simulink model "Torque_controller_MIL"  (R2023b)
settings: Solver=VariableStepAuto  StartTime=0.0  StopTime=15  RelTol=1e-3
values from neighbouring files (symbols this model uses):
  b = 0.016*2.5    (= 0.04)    [torque.m]
  Im = 0.0059*10    (= 0.059)    [torque.m]
  k = kt    (= 1.45433391507)    [torque.m]
  L = 0.0472    [torque.m]
  R = 2.0    (= 2)    [torque.m]
  Ts = 0.005    [torque.m]
libraries: cstblocks x3, simulink x1
settings Model: Creator=giova  LastModifiedBy=david

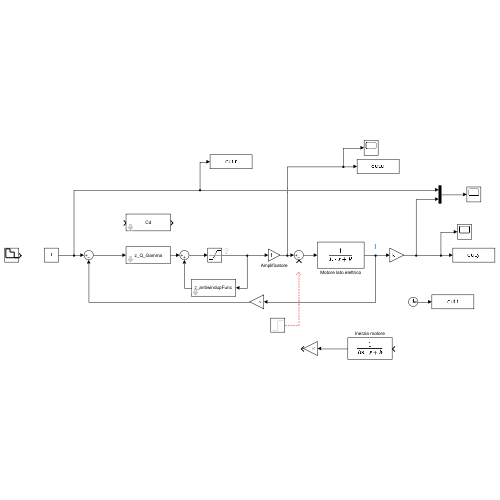
[thumbnail: Simulink's stored preview of the top-level diagram]
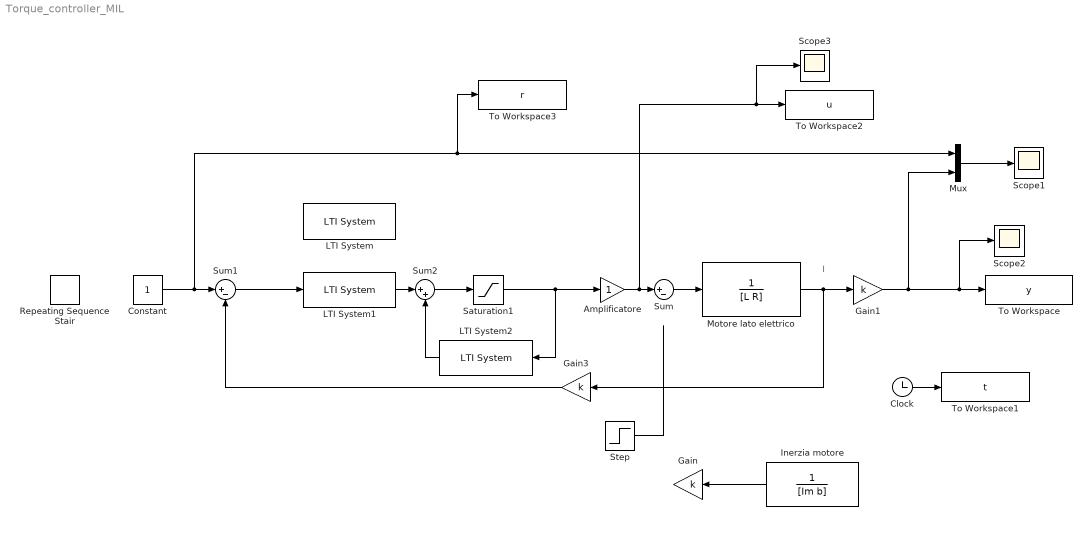
== system Torque_controller_MIL ==
  note: I
  Amplificatore : Gain
  Clock : Clock
  Constant : Constant
  Gain : Gain  Gain=k
  Gain1 : Gain  Gain=k
  Gain3 : Gain  Gain=k
  Inerzia motore : TransferFcn  Denominator=[Im b]
  LTI System : cstblocks/LTI System  sys=Cd  IC=[]  PadeOrder=0
  LTI System1 : cstblocks/LTI System  sys=z_Q_Gamma  IC=[]  PadeOrder=0
  LTI System2 : cstblocks/LTI System  sys=z_antiwindupFunc  IC=[]  PadeOrder=0
  Motore lato elettrico : TransferFcn  Denominator=[L R]
  Mux : Mux  Inputs=2
  Repeating Sequence Stair : simulink/Sources/Repeating Sequence Stair  OutValues=[0.32 0.2 0]  tsamp=5  OutMin=[]  OutMax=[]  OutDataTypeStr=double  OutputDataTypeScalingMode=double  OutDataType=fixdt(0,8)  ConRadixGroup=Best Precision: Vector-wise  OutScaling=2^-12
  Saturation1 : Saturate  UpperLimit=12  LowerLimit=-12
  Scope1 : Scope
  Scope2 : Scope
  Scope3 : Scope
  Step : Step  Time=6  SampleTime=Ts
  Sum : Sum  Inputs=|+-
  Sum1 : Sum  Inputs=|+-
  Sum2 : Sum  Inputs=|++
  To Workspace : ToWorkspace  VariableName=y  SampleTime=-1
  To Workspace1 : ToWorkspace  VariableName=t  SampleTime=-1
  To Workspace2 : ToWorkspace  VariableName=u  SampleTime=-1
  To Workspace3 : ToWorkspace  VariableName=r  SampleTime=-1
  wires:
  Clock/1 -> To Workspace1/1
  Gain1/1 -> Mux/2, Scope2/1, To Workspace/1
  Motore lato elettrico/1 -> Gain1/1, Gain3/1
  Sum/1 -> Motore lato elettrico/1
  Inerzia motore/1 -> Gain/1
  Constant/1 -> To Workspace3/1, Mux/1, Sum1/1
  Mux/1 -> Scope1/1
  Saturation1/1 -> LTI System2/1, Amplificatore/1
  Amplificatore/1 -> Scope3/1, To Workspace2/1, Sum/1
  Gain3/1 -> Sum1/2
  Sum1/1 -> LTI System1/1
  LTI System2/1 -> Sum2/2
  LTI System1/1 -> Sum2/1
  Sum2/1 -> Saturation1/1
  Step/1 -> ?
